simulink model "SensorDataMonitor"  (R2020b)
settings: Solver=FixedStepDiscrete  StartTime=0.0  StopTime=inf  FixedStep=0.01  RelTol=1e-3  EnableMultiTasking=on
values from neighbouring files (symbols this model uses):
  maxAccDiffSum_mg = 0.0    [SensorDataMonitorDD.sldd]
  maxAccVarNoMotion_mg = 250.0    [SensorDataMonitorDD.sldd]
  maxAccVarNoMotionShortTerm_mg = 5.0    [SensorDataMonitorDD.sldd]
  maxDeviationGravityCheck_mg = 300.0    [SensorDataMonitorDD.sldd]
  maxGyrDiffSum_mdegs = 0.0    [SensorDataMonitorDD.sldd]
  maxGyrVarNoMotion_mdegs = 5000.0    [SensorDataMonitorDD.sldd]
  maxGyrVarNoMotionShortTerm_mdegs = 200.0    [SensorDataMonitorDD.sldd]
  maxGyrVarNoMotionSingleAxis_mdegs = 50.0    [SensorDataMonitorDD.sldd]
  maxMeanRotationRate_mdegs = 25000.0    [SensorDataMonitorDD.sldd]
libraries: simulink x4
settings Model: DataDictionary=SensorDataMonitorDD.sldd  EnableAccessToBaseWorkspace=off  DataTypeOverride=Off  DataTypeOverrideAppliesTo=Floating-point  MinMaxOverflowLogging=ForceOff  Creator=stj1si  LastModifiedBy=HNA3SI
settings DataIOCC: SaveFormat=Array  SaveOutput=off  SignalLogging=off  SaveTime=off  ReturnWorkspaceOutputs=off
settings OptimizationCC: DefaultParameterBehavior=Inlined  DefaultUnderspecifiedDataType=single  InlineInvariantSignals=on  EnhancedBackFolding=on  CachingGlobalReferences=on  ExpressionDepthLimit=2147483647  NoFixptDivByZeroProtection=on  EfficientFloat2IntCast=on  LifeSpan=1  MaxStackSize=16384  SimCompilerOptimization=on  EfficientTunableParamExpr=on
settings DebuggingCC: SolverPrmCheckMsg=warning  ParameterPrecisionLossMsg=none  AllowSymbolicDim=off  StateNameClashWarn=warning  SFUnexpectedBacktrackingDiag=warning  SFNoUnconditionalDefaultTransitionDiag=warning  SFExecutionAtInitializationDiag=none  ArithmeticOperatorsInVariantConditions=warning
settings HardwareCC: ProdBitPerPointer=32  ProdBitPerSizeT=32  ProdBitPerPtrDiffT=32  ProdLargestAtomicInteger=Long  ProdLargestAtomicFloat=Double  ProdEndianess=BigEndian  ProdWordSize=32  ProdHWDeviceType=Freescale->32-bit PowerPC
settings ModelReferenceCC: ModelReferenceNumInstancesAllowed=Single  PropagateSignalLabelsOutOfModel=off
settings SFSimCC: SimUseLocalCustomCode=off  MATLABDynamicMemAlloc=off  CustomCodeUndefinedFunction=UseInterfaceOnly
settings RTWCC: Description=Embedded Coder  SystemTargetFile=ert.tlc  GenCodeOnly=on  TemplateMakefile=ert_default_tmf  GenerateReport=on  RTWUseLocalCustomCode=off  IncludeHyperlinkInReport=on  LaunchReport=on  GenerateTraceInfo=on  GenerateTraceReport=on  GenerateTraceReportSl=on  GenerateTraceReportSf=on  GenerateTraceReportEml=on
settings CodeAppCC: IgnoreCustomStorageClasses=off  CustomSymbolStrType=$N$R$M  CustomSymbolStrFcnArg=COCA_rt$I$N$M  CustomSymbolStrBlkIO=COCA_rtb_$N$M  StateflowObjectComments=on  InternalIdentifier=Classic
settings ERTTargetCC: TargetLangStandard=C99 (ISO)  MultiwordLength=2048  GenerateSampleERTMain=on  IncludeMdlTerminateFcn=off  CombineSignalStateStructs=on  SuppressErrorStatus=on  SupportNonFinite=off  SupportComplex=off  CastingMode=Standards  InlinedParameterPlacement=NonHierarchical  ERTSrcFileBannerTemplate=ert_code_template_ebike.cgt  ERTCustomFileTemplate=example_file_process.tlc  ERTFilePackagingFormat=Compact  PreserveExternInFcnDecls=off  SuppressUnreachableDefaultCases=off  EnableSignedLeftShifts=off  EnableSignedRightShifts=off  IndentStyle=Allman  EnableUserReplacementTypes=on
settings ConfigComp: CovEnable=on  CovScope=ReferencedModels  CovIncludeTopModel=off  CovMetricSettings=dw  CovHTMLOptions=-sRT=1 -sVT=0 -aTS=1 -bRG=1 -bTC=1 -hTR=0 -nFC=0 -nFD=1 -scm=1 -bcm=1 -xEv=0 -xEM=0  CovSaveCumulativeToWorkspaceVar=on  CovSaveSingleToWorkspaceVar=on  CovModelRefEnable=all  CovSFcnEnable=off

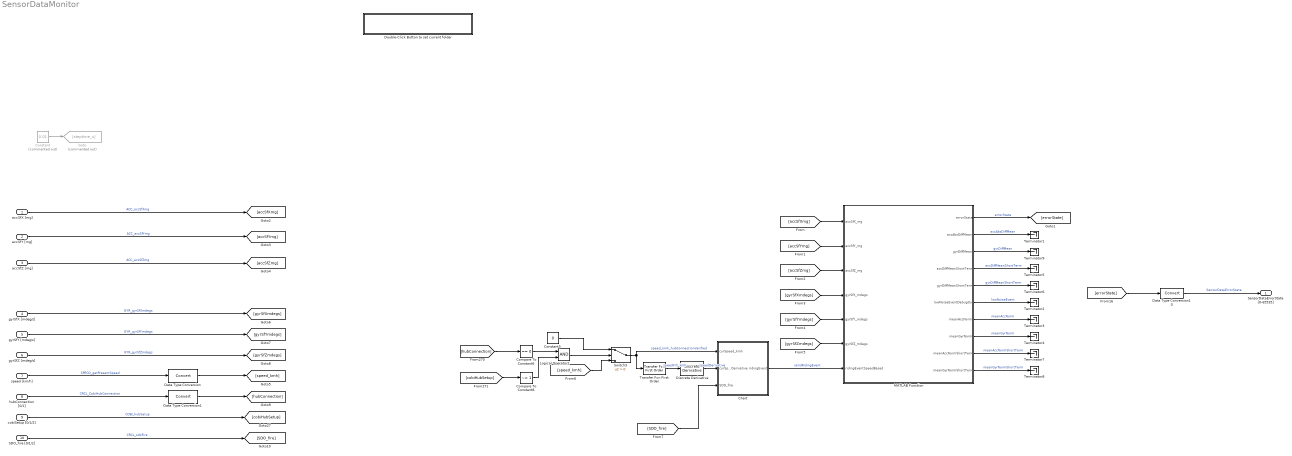
== system SensorDataMonitor ==
  accSfX [mg] : Inport
  accSfY [mg] : Inport  Port=2
  accSfZ [mg] : Inport  Port=3
  gyrSfX [mdeg/s] : Inport  Port=4
  gyrSfY [mdeg/s] : Inport  Port=5
  gyrSfZ [mdeg/s] : Inport  Port=6
  speed [km/h] : Inport  Port=7
  hubConnection [0/1] : Inport  Port=8
  cobiSetup [0/1/2] : Inport  Port=9
  SDO_fire [0/1/2] : Inport  Port=10
  Chart : Stateflow chart  TreatAsAtomicUnit=on
  Compare To Constant6 : simulink/Logic and Bit Operations/Compare To Constant  relop===  const=0  OutDataTypeStr=boolean
  Compare To Constant8 : simulink/Logic and Bit Operations/Compare To Constant  relop=~=  const=1  OutDataTypeStr=boolean
  Constant : Constant  Commented=on  Value=0.01
  Constant5 : Constant  Value=0  OutDataTypeStr=single
  Data Type Conversion : DataTypeConversion
  Data Type Conversion1 : DataTypeConversion
  Data Type Conversion10 : DataTypeConversion  RndMeth=Zero
  Discrete Derivative : simulink/Discrete/Discrete Derivative  gainval=1.0  ICPrevScaledInput=0.0  OutMin=[]  OutMax=[]  OutDataType=fixdt(1, 16)  OutScaling=2^-10  DoSatur=off
  Double-Click Button to set current folder : Subsystem
      settings: OpenFcn=cd(fileparts(get_param(gcs,'filename')));
      mask Display: disp('\bf\fontsize{16}Double-Click to set current folder      ','texmode','on')
  Goto : Goto  Commented=on  GotoTag=steptime_s
  Logical Operator2 : Logic  AllPortsSameDT=off  OutDataTypeStr=boolean
  MATLAB Function : MATLAB Function  TreatAsAtomicUnit=on
  Switch3 : Switch  Criteria=u2 > Threshold
  Terminator{1..9} (9 alike) : Terminator
  Transfer Fcn First Order : simulink/Discrete/Transfer Fcn First Order  PoleZ=0.97  ICPrevOutput=0.0  DoSatur=off
  SensorDataErrorState [0-65535] : Outport  VectorParamsAs1DForOutWhenUnconnected=off
  wires:
  accSfY [mg]/1 -> [accSfYmg]  "ACC_accSfYmg"
  accSfX [mg]/1 -> [accSfXmg]  "ACC_accSfXmg"
  accSfZ [mg]/1 -> [accSfZmg]  "ACC_accSfZmg"
  gyrSfX [mdeg/s]/1 -> [gyrSfXmdegs]  "GYR_gyrSfXmdegs"
  gyrSfY [mdeg/s]/1 -> [gyrSfYmdegs]  "GYR_gyrSfYmdegs"
  gyrSfZ [mdeg/s]/1 -> [gyrSfZmdegs]  "GYR_gyrSfZmdegs"
  Data Type Conversion10/1 -> SensorDataErrorState [0-65535]/1  "SensorDataErrorState"
  Constant/1 -> Goto/1
  [errorState] -> Data Type Conversion10/1
  MATLAB Function/1(errorState) -> [errorState]  "errorState"
  [accSfXmg] -> MATLAB Function/1(accSfX_mg)
  [accSfYmg] -> MATLAB Function/2(accSfY_mg)
  [accSfZmg] -> MATLAB Function/3(accSfZ_mg)
  [gyrSfXmdegs] -> MATLAB Function/4(gyrSfX_mdegs)
  [gyrSfZmdegs] -> MATLAB Function/6(gyrSfZ_mdegs)
  [gyrSfYmdegs] -> MATLAB Function/5(gyrSfY_mdegs)
  MATLAB Function/2(accAbsDiffMean) -> Terminator1/1  "accAbsDiffMean"
  MATLAB Function/6(lowNoiseEventDebugOut) -> Terminator2/1  "lowNoiseEvent"
  MATLAB Function/7(meanAccNorm) -> Terminator3/1  "meanAccNorm"
  MATLAB Function/8(meanGyrNorm) -> Terminator4/1  "meanGyrNorm"
  MATLAB Function/4(accDiffMeanShortTerm) -> Terminator5/1  "accDiffMeanShortTerm"
  MATLAB Function/5(gyrDiffMeanShortTerm) -> Terminator6/1  "gyrDiffMeanShortTerm"
  MATLAB Function/9(meanAccNormShortTerm) -> Terminator7/1  "meanAccNormShortTerm"
  MATLAB Function/10(meanGyrNormShortTerm) -> Terminator8/1  "meanGyrNormShortTerm"
  MATLAB Function/3(gyrDiffMean) -> Terminator9/1  "gyrDiffMean"
  speed [km/h]/1 -> Data Type Conversion/1  "SPECO_getPresentSpeed"
  Chart/1(ridingEvent) -> MATLAB Function/7(ridingEventSpeedBased)  "validRidingEvent"
  Data Type Conversion/1 -> [speed_kmh]
  Data Type Conversion1/1 -> [hubConnection]
  hubConnection [0/1]/1 -> Data Type Conversion1/1  "CRCL_CobiHubConnection"
  Constant5/1 -> Switch3/1
  Compare To Constant8/1 -> Logical Operator2/2
  Switch3/1 -> Transfer Fcn First Order/1, Chart/1(curSpeed_kmh)  "speed_kmh_hubConnectionVerified"
  Logical Operator2/1 -> Switch3/2
  [hubConnection] -> Compare To Constant6/1
  [speed_kmh] -> Switch3/3
  [cobiHubSetup] -> Compare To Constant8/1
  Compare To Constant6/1 -> Logical Operator2/1
  cobiSetup [0/1/2]/1 -> [cobiHubSetup]  "COBI_hubSetup"
  Transfer Fcn First Order/1 -> Discrete Derivative/1  "speedFilt_kmh"
  Discrete Derivative/1 -> Chart/2(curSpeedDerivative)  "speedDerivative"
  SDO_fire [0/1/2]/1 -> [SDO_fire]  "CRCL_sdoFire"
  [SDO_fire] -> Chart/3(SDO_fire)

== system SensorDataMonitor/Double-Click Button to set current folder ==

== matlab function SensorDataMonitor/MATLAB Function ==
  data: accSfX_mg input; errorState output; accAbsDiffMean output; gyrDiffMean output; accDiffMeanShortTerm output; gyrDiffMeanShortTerm output; lowNoiseEventDebugOut output; meanAccNorm output; meanGyrNorm output; meanAccNormShortTerm output; meanGyrNormShortTerm output; accSfY_mg input; accSfZ_mg input; gyrSfX_mdegs input; gyrSfY_mdegs input; gyrSfZ_mdegs input; ridingEventSpeedBased input; maxAccVarNoMotion_mg parameter; maxGyrVarNoMotion_mdegs parameter; maxDeviationGravityCheck_mg parameter; maxMeanRotationRate_mdegs parameter; maxGyrVarNoMotionSingleAxis_mdegs parameter; maxAccDiffSum_mg parameter; maxGyrDiffSum_mdegs parameter; maxGyrVarNoMotionShortTerm_mdegs parameter; maxAccVarNoMotionShortTerm_mg parameter
function [errorState, accAbsDiffMean, gyrDiffMean, ...
    accDiffMeanShortTerm, gyrDiffMeanShortTerm, lowNoiseEventDebugOut, ...
    meanAccNorm, meanGyrNorm, meanAccNormShortTerm, meanGyrNormShortTerm] ...
    = fcn(accSfX_mg, accSfY_mg, accSfZ_mg, ...
    gyrSfX_mdegs, gyrSfY_mdegs, gyrSfZ_mdegs, ridingEventSpeedBased, maxAccVarNoMotion_mg, maxGyrVarNoMotion_mdegs, maxDeviationGravityCheck_mg, maxMeanRotationRate_mdegs, maxGyrVarNoMotionSingleAxis_mdegs, maxAccDiffSum_mg, maxGyrDiffSum_mdegs, maxGyrVarNoMotionShortTerm_mdegs, maxAccVarNoMotionShortTerm_mg)

errorState = uint16(0);

persistent i ringBufFull ringBufAccX ringBufAccY ringBufAccZ ...
    ringBufGyrX ringBufGyrY ringBufGyrZ

if isempty(i)
    i = int16(1);
    ringBufFull = false;
    ringBufAccX = int16(zeros(500,1));
    ringBufAccY = int16(zeros(500,1));
    ringBufAccZ = int16(zeros(500,1));
    ringBufGyrX = int32(zeros(500,1));
    ringBufGyrY = int32(zeros(500,1));
    ringBufGyrZ = int32(zeros(500,1));
end

%fill ringBuffers
ringBufAccX(i) = accSfX_mg;
ringBufAccY(i) = accSfY_mg;
ringBufAccZ(i) = accSfZ_mg;

ringBufGyrX(i) = gyrSfX_mdegs;
ringBufGyrY(i) = gyrSfY_mdegs;
ringBufGyrZ(i) = gyrSfZ_mdegs;

%calculate diff-Vectors
accXDiffVec = diff(ringBufAccX);
accYDiffVec = diff(ringBufAccY);
accZDiffVec = diff(ringBufAccZ);
gyrXDiffVec = abs(diff(ringBufGyrX));
gyrYDiffVec = abs(diff(ringBufGyrY));
gyrZDiffVec = abs(diff(ringBufGyrZ));


%meanDiff
accAbsDiffMean = uint32(mean(abs(accXDiffVec)) + mean(abs(accYDiffVec)) + mean(abs(accZDiffVec)));
gyrDiffMean = uint32(mean(gyrXDiffVec) + mean(gyrYDiffVec) + mean(gyrZDiffVec));

lowNoiseEventDebugOut = uint8(0);
meanGyrNorm = mean(sqrt(single(ringBufGyrX).^2+single(ringBufGyrY).^2+single(ringBufGyrZ).^2));
meanAccNorm = mean(sqrt(single(ringBufAccX).^2+single(ringBufAccY).^2+single(ringBufAccZ).^2));

startSample = int16(0);
shortTermWindowLength = int16(50);
accXDiffVecShortTerm = int16(zeros(shortTermWindowLength,1));
accYDiffVecShortTerm = int16(zeros(shortTermWindowLength,1));
accZDiffVecShortTerm = int16(zeros(shortTermWindowLength,1));
gyrXDiffVecShortTerm = int32(zeros(shortTermWindowLength,1));
gyrYDiffVecShortTerm = int32(zeros(shortTermWindowLength,1));
gyrZDiffVecShortTerm = int32(zeros(shortTermWindowLength,1));
%shortTermMonitor -> last 50 samples

for u=shortTermWindowLength:-1:1
    currentIndex = i - shortTermWindowLength + u;
    if currentIndex <=0
        currentIndex = currentIndex + 500;
    end
    accXDiffVecShortTerm(u) = ringBufAccX(currentIndex);
    accYDiffVecShortTerm(u) = ringBufAccY(currentIndex);
    accZDiffVecShortTerm(u) = ringBufAccZ(currentIndex);
    gyrXDiffVecShortTerm(u) = ringBufGyrX(currentIndex);
    gyrYDiffVecShortTerm(u) = ringBufGyrY(currentIndex);
    gyrZDiffVecShortTerm(u) = ringBufGyrZ(currentIndex);
end

%first estimate shortTerm mean
meanAccNormShortTerm = mean(sqrt(single(accXDiffVecShortTerm).^2+single(accYDiffVecShortTerm).^2+single(accZDiffVecShortTerm).^2));
meanGyrNormShortTerm = mean(sqrt(single(gyrXDiffVecShortTerm).^2+single(gyrYDiffVecShortTerm).^2+single(gyrZDiffVecShortTerm).^2));

%then generate diff shortTerm diff vectors
accXDiffVecShortTerm = abs(diff(accXDiffVecShortTerm));
accYDiffVecShortTerm = abs(diff(accYDiffVecShortTerm));
accZDiffVecShortTerm = abs(diff(accZDiffVecShortTerm));
gyrXDiffVecShortTerm = abs(diff(gyrXDiffVecShortTerm));
gyrYDiffVecShortTerm = abs(diff(gyrYDiffVecShortTerm));
gyrZDiffVecShortTerm = abs(diff(gyrZDiffVecShortTerm));

% if i <= shortTermWindowLength
%     startSample = int16(i) - shortTermWindowLength + 500;
%     accXDiffVecShortTerm = abs(diff([ringBufAccX(startSample:500);ringBufAccX(1:i)]));
%     accYDiffVecShortTerm = abs(diff([ringBufAccY(startSample:500);ringBufAccY(1:i)]));
%     accZDiffVecShortTerm = abs(diff([ringBufAccZ(startSample:500);ringBufAccZ(1:i)]));
%     gyrXDiffVecShortTerm = abs(diff([ringBufGyrX(startSample:500);ringBufGyrX(1:i)]));
%     gyrYDiffVecShortTerm = abs(diff([ringBufGyrY(startSample:500);ringBufGyrY(1:i)]));
%     gyrZDiffVecShortTerm = abs(diff([ringBufGyrZ(startSample:500);ringBufGyrZ(1:i)]));
%     meanGyrNormShortTerm = mean(sqrt(single([ringBufGyrX(startSample:500);ringBufGyrX(1:i)]).^2+single([ringBufGyrY(startSample:500);ringBufGyrY(1:i)]).^2+single([ringBufGyrZ(startSample:500);ringBufGyrZ(1:i)]).^2));
%     meanAccNormShortTerm = mean(sqrt(single([ringBufAccX(startSample:500);ringBufAccX(1:i)]).^2+single([ringBufAccY(startSample:500);ringBufAccY(1:i)]).^2+single([ringBufAccZ(startSample:500);ringBufAccZ(1:i)]).^2));
% else
%     startSample = int16(i) - shortTermWindowLength;
%     accXDiffVecShortTerm = abs(diff(ringBufAccX(startSample:i)));
%     accYDiffVecShortTerm = abs(diff(ringBufAccY(startSample:i)));
%     accZDiffVecShortTerm = abs(diff(ringBufAccZ(startSample:i)));
%     gyrXDiffVecShortTerm = abs(diff(ringBufGyrX(startSample:i)));
%     gyrYDiffVecShortTerm = abs(diff(ringBufGyrY(startSample:i)));
%     gyrZDiffVecShortTerm = abs(diff(ringBufGyrZ(startSample:i)));
%     meanGyrNormShortTerm = mean(sqrt(single(ringBufGyrX(startSample:i)).^2+single(ringBufGyrY(startSample:i)).^2+single(ringBufGyrZ(startSample:i)).^2));
%     meanAccNormShortTerm = mean(sqrt(single(ringBufAccX(startSample:i)).^2+single(ringBufAccY(startSample:i)).^2+single(ringBufAccZ(startSample:i)).^2));
% end

accDiffMeanShortTerm = uint32(mean(accXDiffVecShortTerm) + mean(accYDiffVecShortTerm) + mean(accZDiffVecShortTerm));
gyrDiffMeanShortTerm = uint32(mean(gyrXDiffVecShortTerm) + mean(gyrYDiffVecShortTerm) + mean(gyrZDiffVecShortTerm));

if ringBufFull
    %acc variance check
    if sum(abs(accXDiffVec)) <= maxAccDiffSum_mg
        errorState = errorState + 1;
    end
    if sum(abs(accYDiffVec)) <= maxAccDiffSum_mg
        errorState = errorState + 2;
    end
    if sum(abs(accZDiffVec)) <= maxAccDiffSum_mg
        errorState = errorState + 4;
    end
    
    %gyr variance check
    if sum(gyrXDiffVec) <= maxGyrDiffSum_mdegs
        errorState = errorState + 8;
    end
    if sum(gyrYDiffVec) <= maxGyrDiffSum_mdegs
        errorState = errorState + 16;
    end
    if sum(gyrZDiffVec) <= maxGyrDiffSum_mdegs
        errorState = errorState + 32;
    end
    
    %lowVarianceSituation
    %ShortTerm   
    if accDiffMeanShortTerm < maxAccVarNoMotionShortTerm_mg && gyrDiffMeanShortTerm < maxGyrVarNoMotionShortTerm_mdegs
        lowNoiseEventDebugOut = uint8(1);
        %acc 1 g norm check
        if abs(1000-meanAccNormShortTerm) > maxDeviationGravityCheck_mg 
            errorState = errorState + 64;
        end
        
        %gyr 0 °/s norm check
        if meanGyrNormShortTerm > maxMeanRotationRate_mdegs 
            errorState = errorState + 128;
        end
        
    %LongTerm    
    elseif accAbsDiffMean < maxAccVarNoMotion_mg && gyrDiffMean < maxGyrVarNoMotion_mdegs
        lowNoiseEventDebugOut = uint8(2);
        %acc 1 g norm check
        if abs(1000-meanAccNorm) > maxDeviationGravityCheck_mg  % && (mean(accXDiffVec) < 5 || mean(accYDiffVec) < 5 || mean(accZDiffVec) < 5)
            errorState = errorState + 64;
        end
        
        %gyr 0 °/s norm check
        if meanGyrNorm > maxMeanRotationRate_mdegs && ...
                (mean(gyrXDiffVec) < maxGyrVarNoMotionSingleAxis_mdegs || ...
                mean(gyrYDiffVec) < maxGyrVarNoMotionSingleAxis_mdegs || ...
                mean(gyrZDiffVec) < maxGyrVarNoMotionSingleAxis_mdegs)
            errorState = errorState + 128;
        end
    end    
    
    %highSpeed but low acc and gyr variance
    if accAbsDiffMean < 10 && gyrDiffMean < 500 && ...
            ridingEventSpeedBased == true 
        errorState = errorState + 256;
    end
end

%reset ringBuf Counter
if i >= 500
    i = int16(1);
    % when ringBuffer is filled for the first time, sensor checks can be
    % started
    if ringBufFull == false
        ringBufFull = true;
    end
else
    i = i + 1;
end

end

== stateflow chart SensorDataMonitor/Chart ==
  state speed
    en:
  state Idle
    en:
    ridingEvent = false;
  state validSpeedEvent
    en:
    ridingEvent = true;
  (default) -> Idle
  Idle -> speed : [curSpeed_kmh > 10]
  speed -> Idle [order 1] : [curSpeed_kmh < 5 || SDO_fire >= 1]
  speed -> validSpeedEvent [order 2] : %positive speedDerivative to prevent rotating backwheels of rolledOver eBikes
      | [after(5,sec) && ...
      | curSpeedDerivative > 0]
  validSpeedEvent -> Idle [order 1] : [curSpeed_kmh < 5 || SDO_fire >= 1 || ...
      | (after(5,sec) && curSpeedDerivative < -1) || ... % only decreasing speed -> rotating backWheel of rollOVer eBike
      | (after(10,sec) && curSpeedDerivative <= 0.001)... % constant speed -> no validSpeedEvent
      | ]
  validSpeedEvent -> validSpeedEvent [order 2] : [curSpeedDerivative > 0.01]
  data: curSpeed_kmh input single; ridingEvent output boolean; curSpeedDerivative input; SDO_fire input
